simulink model "modelloTC_es1_sol2"  (R2021a)
settings: Solver=ode23  StartTime=0.0  StopTime=10.0  RelTol=1e-3
values from neighbouring files (symbols this model uses):
  f = sym('f')    [fdt_es1.m]
  g = sym('g')    [fdt_es1.m]
  k = sym('k')    [fdt_es1.m]
  M1 = sym('M1')    [fdt_es1.m]
  M2 = sym('M2')    [fdt_es1.m]
settings Model: Creator=User_LABORATORIO  LastModifiedBy=User_LABORATORIO

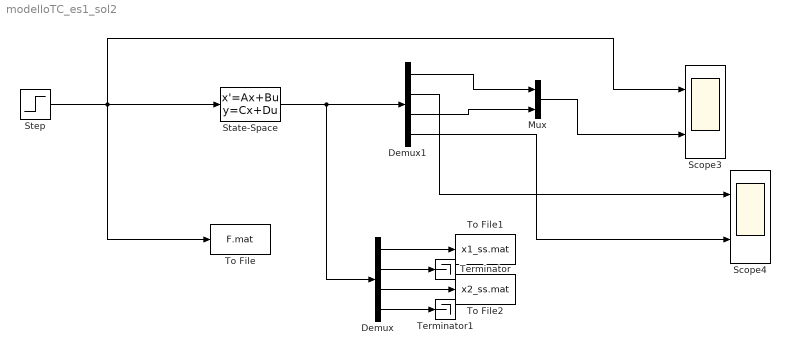
== system modelloTC_es1_sol2 ==
  Demux : Demux
  Demux1 : Demux
  Mux : Mux  Inputs=2
  Scope3 : Scope  NumInputPorts=2
  Scope4 : Scope  NumInputPorts=2
  State-Space : StateSpace  A=[0 1 0 0;-k/M1 -g*f k/M1 0;0 0 0 1;k/M2 0 -k/M2 -g*f]  B=[0;1/M1;0;0]  C=[1 0 0 0; 0 1 0 0;0 0 1 0;0 0 0 1]  D=[0;0;0;0]  InitialCondition=0
  Step : Step  SampleTime=0
  Terminator : Terminator
  Terminator1 : Terminator
  To File : ToFile  Filename=F.mat  SaveFormat=Timeseries
  To File1 : ToFile  Filename=x1_ss.mat  SaveFormat=Timeseries
  To File2 : ToFile  Filename=x2_ss.mat  SaveFormat=Timeseries
  wires:
  Demux/4 -> Terminator1/1
  Demux/2 -> Terminator/1
  State-Space/1 -> Demux/1, Demux1/1
  Demux/3 -> To File2/1
  Demux1/1 -> Mux/1
  Demux1/2 -> Scope4/1
  Mux/1 -> Scope3/2
  Step/1 -> To File/1, Scope3/1, State-Space/1
  Demux/1 -> To File1/1
  Demux1/4 -> Scope4/2
  Demux1/3 -> Mux/2
